simulink model "plant"  (R2024a)
settings: Solver=VariableStepAuto  StartTime=0.0  StopTime=10.0  RelTol=1e-3
values from neighbouring files (symbols this model uses):
  A_air = 0.00588710854841    [run1.mat]    (also in run2.mat)
  Cs = 0.9    [run1.mat]    (also in run2.mat)
  h = 0.0127000254001    [run1.mat]    (also in run2.mat)
  m = 100    [run1.mat]    (also in run2.mat)
  T_f = 21    [run1.mat]    (also in run2.mat)
settings Model: Creator=veswaranandam  LastModifiedBy=veswaranandam

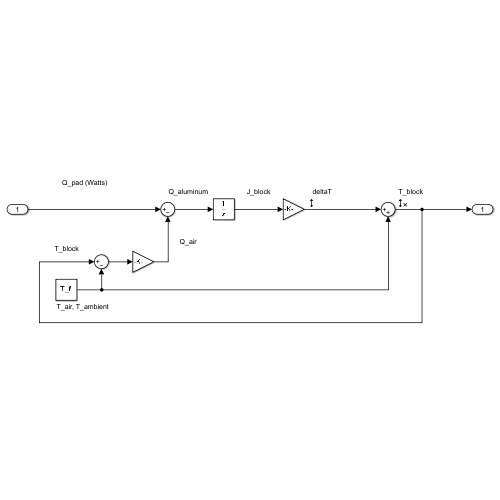
[thumbnail: Simulink's stored preview of the top-level diagram]
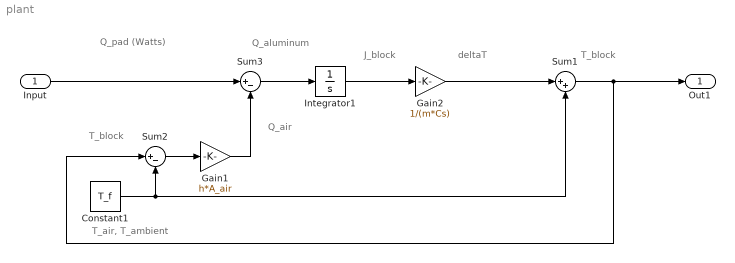
== system plant ==
  note: J_block
  note: Q_pad (Watts)
  note: T_block
  note: T_block
  note: Q_air
  note: Q_aluminum
  note: deltaT
  note: T_air, T_ambient
  Input : Inport
  Constant1 : Constant  Value=T_f
  Gain1 : Gain  Gain=h*A_air
  Gain2 : Gain  Gain=1/(m*Cs)
  Integrator1 : Integrator
  Sum1 : Sum  Inputs=|++
  Sum2 : Sum  Inputs=|+-
  Sum3 : Sum  Inputs=|+-
  Out1 : Outport
  wires:
  Integrator1/1 -> Gain2/1
  Sum1/1 -> Out1/1, Sum2/1
  Gain2/1 -> Sum1/1
  Sum3/1 -> Integrator1/1
  Sum2/1 -> Gain1/1
  Gain1/1 -> Sum3/2
  Constant1/1 -> Sum1/2, Sum2/2
  Input/1 -> Sum3/1
